simulink model "Hierarchy4_tmp"  (Simulink 8.3)
settings: Solver=ode45  StartTime=0.0  StopTime=10.0  RelTol=1e-3
settings Model: Creator=scaife  LastModifiedBy=bourbouh  CovSFcnEnable=on  ExtModeAutoUpdateStatusClock=off
settings DataIOCC: SignalLoggingName=sigsOut
settings DebuggingCC: SaveWithParameterizedLinksMsg=none  SignalResolutionControl=TryResolveAllWithWarning  SolverPrmCheckMsg=none  MultiTaskDSMMsg=warning  MultiTaskCondExecSysMsg=none  FrameProcessingCompatibilityMsg=error  StateNameClashWarn=none
settings HardwareCC: TargetUnknown=on
settings SFSimCC: SimParseCustomCode=off
settings GRTTargetCC: GeneratePreprocessorConditionals=Use local settings

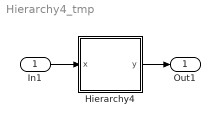
== system Hierarchy4_tmp ==
  In1 : Inport
  Hierarchy4 : Stateflow chart  TreatAsAtomicUnit=on
      settings: PermitHierarchicalResolution=ParametersOnly
  Out1 : Outport
  wires:
  In1/1 -> Hierarchy4/1(x)
  Hierarchy4/1(y) -> Out1/1

== stateflow chart Hierarchy4 ==
  state A/
    en: y=1;
  state B/
    en: y=2;
  (default) -> A [order 1] : [x==0]
  (default) -> B [order 2] : [x<>0]
  data: x input int32; y output int32
